simulink model "furnace_emul_v12"  (Simulink 5.0)
settings: Solver=FixedStepDiscrete  StartTime=0.0  StopTime=9000  RelTol=1e-3
values from neighbouring files (symbols this model uses):
  A_amb = pi*(D_e+2*d_ins)*L    (= 0.0498884492)    [tube_ini.m]
  A_e = pi*D_e*L    (= 0.0247557292)    [tube_ini.m]
  A_pi = pi*D_pi*L    (= 0.017592904)    [tube_ini.m]
  A_po = pi*D_po*L    (= 0.0184725492)    [tube_ini.m]
  A_w = pi/4*D_w^2*n_sl    (= 0.0628318)    [tube_ini.m]
  A_wc = pi*D_w*Li    (= 0.01256636)    [tube_ini.m]
  D_pi = D_w+2*DX_R    (= 0.28)    [tube_ini.m]
  D_w = 0.2    [tube_ini.m]
  elem_tmax = 1250    [tube_ini.m]
  F_A_e = lam_p_bct*F_A_e+lam_p_bcb*F_A_e([n:-1:1])    [tube_ini.m]
  F_A_ew = e_ew*A_ew./((1/ei-1)+(1/eo-1)*D_pi/D_w+1./(toeplitz(F1*Li)))    [tube_ini.m]
  F_A_p = lam_p_bct*F_A_p+lam_p_bcb*F_A_p([n:-1:1])    [tube_ini.m]
  F_A_pe = A_ep./((1/ei-1)+(1/eo-1)*D_po/D_e+1./(toeplitz(F1*Li)))    [tube_ini.m]
  F_A_pw = A_pw./((1/ei-1)+(1/eo-1)*D_pi/D_w+1./(toeplitz(F1*Li)))    [tube_ini.m]
  f_amb_ped = 1    [tube_ini.m]
  f_amb_top = .3    (= 0.3)    [tube_ini.m]
  Fb_A_ew = e_ew*Aib./((1/ei-1)+(1/eo-1)*Aib/A+1./(F4*Li))    [tube_ini.m]
  Fb_A_pw = Aib./((1/ei-1)+(1/eo-1)*Aib/A+1./(F4*Li))    [tube_ini.m]
  Fs_e = e_ew*A_e./((1/eo-1)+(1/eo-1)+1./(toeplitz(F5*Li)))    [tube_ini.m]
  Fs_p = A_pi./((1/eo-1)+(1/eo-1)+1./(toeplitz(F5*Li)))    [tube_ini.m]
  gww_bot = ones(N_w,1)*SW    [tube_ini.m]
  gww_top = gww_bot    [tube_ini.m]
  h_amb = 1    [tube_ini.m]
  h_gas = 2    [tube_ini.m]
  H_Z = zeros(n,5)    [tube_ini.m]
  k_adj_ped = 0.6    [tube_ini.m]
  k_adj_top = 0.5    [tube_ini.m]
  L = 0.2    [M_Hist040407.m]    (also in exp303.m = 500:499+ly; tube_ini.m = 0.02)
  lam_p_bcb = 1    [tube_ini.m]
  lam_p_bct = .4    (= 0.4)    [tube_ini.m]
  Li = dx_w    (= 0.02)    [tube_ini.m]
  m_e = rho_e*V_e    (= 0.6312710946)    [tube_ini.m]
  m_p = V_p*rho_p    (= 0.30294980688)    [tube_ini.m]
  m_ped = V_ped*rho_p    (= 1.5079632)    [tube_ini.m]
  m_top = rho_p*V_top    (= 1.5079632)    [tube_ini.m]
  m_w = rho_w*V_w    (= 0.146398094)    [tube_ini.m]
  mcp_adj_ped = 0.36    [tube_ini.m]
  mcp_adj_top = 0.25    [tube_ini.m]
  n = N_w+N_top+N_ped    [tube_ini.m]
  N_ped = round(DX_P/Li)    [tube_ini.m]
  N_top = n-N_w-N_p    [s_tubew.m]    (also in tube_ini.m = round(DX_T/Li))
  N_w = 100/n_sl    (= 50)    [tube_ini.m]
  pow_pm = pow_pml*pi*D_e*n*L/(d_e+d_g)    [tube_ini.m]
  pr_gas = 0.2    [tube_ini.m]
  PRG = 0*SPE; for ii=1:length(profile_loc); PRG(ii,profile_loc(ii))=1;end    [tube_ini.m]
  profile_loc = [N_top,h_zones(1)+round(h_zones(2)/2),   sum(h_zones(1:2))+round(h_zones(3)/2),sum(h_zones(1:3))+round(h_zones(4)/2),   n-N_ped]    [tube_ini.m]
  PRT = PRT'    [tube_ini.m]
  PRW = PRW'    [tube_ini.m]
  SPE = SPE'    [tube_ini.m]
  spike_loc = [round(h_zones(1)/2),h_zones(1)+round(h_zones(2)/2),   sum(h_zones(1:2))+round(h_zones(3)/2),sum(h_zones(1:3))+round(h_zones(4)/2),   sum(h_zones(1:4))+round(h_zones(5)/2)]    [tube_ini.m]
  SPT = SPT'    [tube_ini.m]
  T_0 = T_01*ones(n,1)    [tube_ini.m]
  T_a0 = T_a01*ones(n,1)    [tube_ini.m]
  T_amb = 25    [tube_ini.m]
  T_w0 = T_amb*ones(N_w,1)    [tube_ini.m]
  T_w0_ped = T_amb*ones(N_ped,1)    [tube_ini.m]
  T_w0_top = T_01*ones(N_top,1)    [tube_ini.m]
  Tsa = .5    (= 0.5)    [tube_ini.m]
  tube_tmax = 1200    [tube_ini.m]
  V_a = pi/4*D_pi^2*L    (= 0.00123150328)    [tube_ini.m]
undefined symbols (not defined in the file or in its folder): N, s_tubew
libraries: simulink3 x19, simulink x2
(part 2 of 2)

== system furnace_emul_v12/Furnace Emulator v1.2/Heat Exchange/gas-waf_exch/i-i convection ==
  ta_t0 : Inport
  tw : Inport  Port=2
  Index : Inport  Port=3
  A : Inport  Port=4
  Assignment : Assignment  ElementSrc=External
  Assignment1 : Assignment  ElementSrc=External
  Proportional2 : Gain  Gain=0  SaturateOnIntegerOverflow=on
  Selector1 : Selector  ElementSrc=External  Elements=[1:n]  InputPortWidth=n*2
  Selector3 : Selector  Elements=[1:n]  InputPortWidth=n*2
  convection1 : Subsystem
  dh_a : Outport
  dh_w : Outport  Port=2
  wires:
  Index/1 -> Assignment/3, Selector1/2, Assignment1/3
  Assignment/1 -> convection1/2(T+)
  ta_t0/1 -> convection1/1(T-), Assignment/1, Proportional2/1
  tw/1 -> Assignment/2
  Selector1/1 -> dh_w/1
  convection1/1(Out1) -> Selector3/1, Selector1/1
  Selector3/1 -> dh_a/1
  Assignment1/1 -> convection1/3(A)
  Proportional2/1 -> Assignment1/1
  A/1 -> Assignment1/2

== system furnace_emul_v12/Furnace Emulator v1.2/Heat Exchange/gas-waf_exch/i-i convection1 ==
  ta_t0 : Inport
  tw : Inport  Port=2
  Index : Inport  Port=3
  A : Inport  Port=4
  Assignment : Assignment  ElementSrc=External
  Assignment1 : Assignment  ElementSrc=External
  Proportional2 : Gain  Gain=0  SaturateOnIntegerOverflow=on
  Selector1 : Selector  ElementSrc=External  Elements=[1:n]  InputPortWidth=n*2
  Selector3 : Selector  Elements=[1:n]  InputPortWidth=n*2
  convection1 : Subsystem
  dh_a : Outport
  dh_w : Outport  Port=2
  wires:
  A/1 -> Assignment1/2
  Proportional2/1 -> Assignment1/1
  Assignment1/1 -> convection1/3(A)
  Selector3/1 -> dh_a/1
  convection1/1(Out1) -> Selector1/1, Selector3/1
  Selector1/1 -> dh_w/1
  tw/1 -> Assignment/2
  ta_t0/1 -> Proportional2/1, Assignment/1, convection1/1(T-)
  Assignment/1 -> convection1/2(T+)
  Index/1 -> Assignment1/3, Selector1/2, Assignment/3

== system furnace_emul_v12/Furnace Emulator v1.2/Heat Exchange/prof-waf_xch/waf_rad ==
  Tp+ : Inport  Orientation=left
  Tw- : Inport  Orientation=left  Port=2
  nw0 : Inport  Port=3
  Constant1 : Constant  Value=ones(1,2*n)  VectorParams1D=off
  Constant2 : Constant  Value=ones(2*n,1)  VectorParams1D=off
  MATLAB Fcn : MATLABFcn  MATLABFcn=s_tubew(u,n,N_w,N_ped,F_A_pw,Fb_A_pw,Fs_p)  OutputDimensions=[2*n,2*n]  Output1D=off
  Product : Product  SaturateOnIntegerOverflow=on  InputSameDT=on
  Product{1..4} (4 alike) : Product  Multiplication=Matrix(*)  SaturateOnIntegerOverflow=on  InputSameDT=on
  Reshape : simulink3/Signals & Systems/Reshape  OutputDimensionality=Column vector  OutputDimensions=[N,N_w]
  Reshape1 : simulink3/Signals & Systems/Reshape  OutputDimensionality=Row vector  OutputDimensions=[N,N_w]
  Reshape2 : simulink3/Signals & Systems/Reshape  OutputDimensionality=1-D array  OutputDimensions=[N,N_w]
  Reshape3 : simulink3/Signals & Systems/Reshape  OutputDimensionality=1-D array  OutputDimensions=[N,N_w]
  elem_prof_rad : Subsystem
  dh+ : Outport  Orientation=left
  dh- : Outport  Orientation=left  Port=2
  wires:
  nw0/1 -> MATLAB Fcn/1
  Constant1/1 -> Product1/2, Product4/1
  Reshape/1 -> Product1/1
  Constant2/1 -> Product3/2, Product2/1
  Reshape1/1 -> Product2/2
  Product1/1 -> elem_prof_rad/1(T+)
  Product2/1 -> elem_prof_rad/2(T-)
  MATLAB Fcn/1 -> Product/1
  elem_prof_rad/1(DTH) -> Product/2
  Product/1 -> Product3/1, Product4/2
  Product3/1 -> Reshape2/1
  Product4/1 -> Reshape3/1
  Tp+/1 -> Reshape/1
  Tw-/1 -> Reshape1/1
  Reshape3/1 -> dh-/1
  Reshape2/1 -> dh+/1

== system furnace_emul_v12/Furnace Emulator v1.2/Heat Exchange/profile/amb_prof_rad ==
  T+ : Inport
  T- : Inport  Port=2
  Constant1 : Constant  Value=4
  Constant2 : Constant  Value=273
  Constant3 : Constant  Value=4
  Constant4 : Constant  Value=273
  Math Function : Math  Operator=pow
  Math Function1 : Math  Operator=pow
  Proportional1 : Gain  Gain=5.675  SaturateOnIntegerOverflow=on
  Proportional3 : Gain  Gain=0.01  SaturateOnIntegerOverflow=on
  Proportional4 : Gain  Gain=0.01  SaturateOnIntegerOverflow=on
  Sum1 : Sum  Inputs=2  SaturateOnIntegerOverflow=on  InputSameDT=on
  Sum2 : Sum  Inputs=2  SaturateOnIntegerOverflow=on  InputSameDT=on
  Sum3 : Sum  Inputs=+-  SaturateOnIntegerOverflow=on  InputSameDT=on
  DTH : Outport
  wires:
  Sum3/1 -> Proportional1/1
  Proportional1/1 -> DTH/1
  Math Function1/1 -> Sum3/2
  Math Function/1 -> Sum3/1
  T-/1 -> Sum1/1
  Constant4/1 -> Sum1/2
  Sum1/1 -> Proportional4/1
  Proportional4/1 -> Math Function1/1
  Constant3/1 -> Math Function1/2
  T+/1 -> Sum2/1
  Constant2/1 -> Sum2/2
  Sum2/1 -> Proportional3/1
  Proportional3/1 -> Math Function/1
  Constant1/1 -> Math Function/2

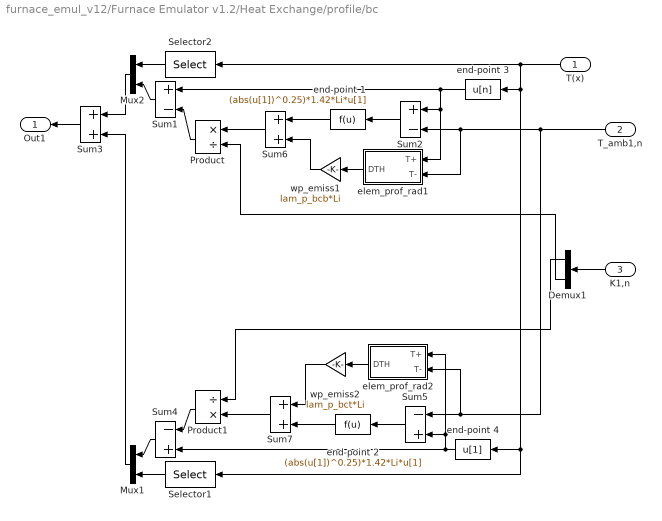
== system furnace_emul_v12/Furnace Emulator v1.2/Heat Exchange/profile/bc ==
  T(x) : Inport  Orientation=left
  T_amb1,n : Inport  Orientation=left  Port=2
  K1,n : Inport  Orientation=left  Port=3
  Demux1 : Demux  Orientation=left  Outputs=2
  Mux1 : Mux  Orientation=left  Inputs=2
  Mux2 : Mux  Orientation=left  Inputs=2
  Product : Product  Orientation=left  Inputs=*/  SaturateOnIntegerOverflow=on  InputSameDT=on
  Product1 : Product  Orientation=left  Inputs=/*  SaturateOnIntegerOverflow=on  InputSameDT=on
  Selector1 : Selector  Orientation=left  Elements=[1:n-1]  InputPortWidth=n
  Selector2 : Selector  Orientation=left  Elements=[2:n]  InputPortWidth=n
  Sum1 : Sum  Orientation=left  Inputs=+-  SaturateOnIntegerOverflow=on  InputSameDT=on
  Sum2 : Sum  Orientation=left  Inputs=+-  SaturateOnIntegerOverflow=on  InputSameDT=on
  Sum3 : Sum  Orientation=left  Inputs=2  SaturateOnIntegerOverflow=on  InputSameDT=on
  Sum4 : Sum  Orientation=left  Inputs=-+  SaturateOnIntegerOverflow=on  InputSameDT=on
  Sum5 : Sum  Orientation=left  Inputs=-+  SaturateOnIntegerOverflow=on  InputSameDT=on
  Sum6 : Sum  Orientation=left  Inputs=2  SaturateOnIntegerOverflow=on  InputSameDT=on
  Sum7 : Sum  Orientation=left  Inputs=2  SaturateOnIntegerOverflow=on  InputSameDT=on
  elem_prof_rad1 : Subsystem  Orientation=left
  elem_prof_rad2 : Subsystem  Orientation=left
  end-point 1 : Fcn  Orientation=left  Expr=(abs(u[1])^0.25)*1.42*Li*u[1]
  end-point 2 : Fcn  Orientation=left  Expr=(abs(u[1])^0.25)*1.42*Li*u[1]
  end-point 3 : Fcn  Orientation=left  Expr=u[n]
  end-point 4 : Fcn  Orientation=left  Expr=u[1]
  wp_emiss1 : Gain  Orientation=left  Gain=lam_p_bcb*Li  SaturateOnIntegerOverflow=on
  wp_emiss2 : Gain  Orientation=left  Gain=lam_p_bct*Li  SaturateOnIntegerOverflow=on
  Out1 : Outport  Orientation=left
  wires:
  Demux1/1 -> Product1/1
  Product1/1 -> Sum4/1
  Demux1/2 -> Product/2
  Product/1 -> Sum1/2
  K1,n/1 -> Demux1/1
  Selector2/1 -> Mux2/1
  Selector1/1 -> Mux1/2
  T(x)/1 -> Selector2/1, end-point 3/1, end-point 4/1, Selector1/1
  Mux1/1 -> Sum3/2
  Mux2/1 -> Sum3/1
  Sum3/1 -> Out1/1
  Sum1/1 -> Mux2/2
  end-point 3/1 -> Sum1/1, Sum2/1, elem_prof_rad1/1(T+)
  Sum2/1 -> end-point 1/1
  Sum4/1 -> Mux1/1
  end-point 4/1 -> Sum4/2, Sum5/2, elem_prof_rad2/1(T+)
  Sum5/1 -> end-point 2/1
  T_amb1,n/1 -> Sum2/2, elem_prof_rad1/2(T-), Sum5/1, elem_prof_rad2/2(T-)
  elem_prof_rad1/1(DTH) -> wp_emiss1/1
  Sum6/1 -> Product/1
  end-point 1/1 -> Sum6/1
  wp_emiss1/1 -> Sum6/2
  elem_prof_rad2/1(DTH) -> wp_emiss2/1
  end-point 2/1 -> Sum7/2
  wp_emiss2/1 -> Sum7/1
  Sum7/1 -> Product1/2

== system furnace_emul_v12/Furnace Emulator v1.2/Heat Exchange/wafer/Top plate ==
  heat In1 : Inport
  amb : Inport  Orientation=left  Port=2
  Constant1 : Constant  Orientation=left  Value=mcp_adj_top
  Constant2 : Constant  Orientation=left  Value=k_adj_top
  Discrete-Time Integrator : DiscreteIntegrator  InitialCondition=T_w0_top  SampleTime=Tsa
  Product : Product  Inputs=*//  SaturateOnIntegerOverflow=on  InputSameDT=on
  Product1 : Product  Inputs=3  SaturateOnIntegerOverflow=on  InputSameDT=on
  Proportional12 : Gain  Orientation=left  Gain=V_top/Li/Li  SaturateOnIntegerOverflow=on
  Proportional2 : Gain  Gain=1/m_top  SaturateOnIntegerOverflow=on
  Proportional7 : Gain  Orientation=left  Gain=2  SaturateOnIntegerOverflow=on
  Selector1 : Selector  Orientation=left  Elements=[1]  InputPortWidth=N_top
  Sum2 : Sum  SaturateOnIntegerOverflow=on  InputSameDT=on
  Sum7 : Sum  Orientation=left  Inputs=-+  SaturateOnIntegerOverflow=on  InputSameDT=on
  bc : Subsystem  Orientation=left
  cp Look-Up Table : Lookup  Orientation=left  InputValues=[400, 600, 800, 1000, 1200]-273  OutputValues=[790 867 913 946 967]  SaturateOnIntegerOverflow=on
  k Look-Up Table : Lookup  Orientation=left  InputValues=[400, 600, 800, 1300]-273  OutputValues="[7.6  5  4.2  3.2 ]"  SaturateOnIntegerOverflow=on
  Ti(x) : Outport
  wires:
  Discrete-Time Integrator/1 -> cp Look-Up Table/1, Ti(x)/1, Proportional7/1, bc/1(T(x)), k Look-Up Table/1
  Sum2/1 -> Proportional2/1
  Product/1 -> Discrete-Time Integrator/1
  Proportional2/1 -> Product/1
  cp Look-Up Table/1 -> Product/2
  heat In1/1 -> Sum2/1
  k Look-Up Table/1 -> Selector1/1, Product1/1
  Selector1/1 -> bc/3(K,1)
  Sum7/1 -> Proportional12/1
  bc/1(Out1) -> Sum7/2
  Proportional7/1 -> Sum7/1
  amb/1 -> bc/2(T_amb1)
  Product1/1 -> Sum2/2
  Proportional12/1 -> Product1/2
  Constant1/1 -> Product/3
  Constant2/1 -> Product1/3

== system furnace_emul_v12/Furnace Emulator v1.2/Heat Exchange/wafer/pedestal ==
  heat In1 : Inport
  Tamb_b : Inport  Orientation=left  Port=2
  Constant1 : Constant  Orientation=left  Value=mcp_adj_ped
  Constant2 : Constant  Orientation=left  Value=k_adj_ped
  Discrete-Time Integrator : DiscreteIntegrator  InitialCondition=T_w0_ped  SampleTime=Tsa
  Product : Product  Inputs=*//  SaturateOnIntegerOverflow=on  InputSameDT=on
  Product1 : Product  Inputs=3  SaturateOnIntegerOverflow=on  InputSameDT=on
  Proportional12 : Gain  Orientation=left  Gain=V_ped/Li/Li  SaturateOnIntegerOverflow=on
  Proportional2 : Gain  Gain=1/m_ped  SaturateOnIntegerOverflow=on
  Proportional7 : Gain  Orientation=left  Gain=2  SaturateOnIntegerOverflow=on
  Selector1 : Selector  Orientation=left  Elements=[N_ped]  InputPortWidth=N_ped
  Sum2 : Sum  SaturateOnIntegerOverflow=on  InputSameDT=on
  Sum7 : Sum  Orientation=left  Inputs=-+  SaturateOnIntegerOverflow=on  InputSameDT=on
  bc : Subsystem  Orientation=left
  cp Look-Up Table : Lookup  Orientation=left  InputValues=[400, 600, 800, 1000, 1200]-273  OutputValues=[790 867 913 946 967]  SaturateOnIntegerOverflow=on
  k Look-Up Table : Lookup  Orientation=left  InputValues=[400, 600, 800, 1300]-273  OutputValues="[7.6  5  4.2  3.2 ]"  SaturateOnIntegerOverflow=on
  Ti(x) : Outport
  wires:
  heat In1/1 -> Sum2/1
  cp Look-Up Table/1 -> Product/2
  Proportional2/1 -> Product/1
  Product/1 -> Discrete-Time Integrator/1
  Sum2/1 -> Proportional2/1
  Discrete-Time Integrator/1 -> cp Look-Up Table/1, Ti(x)/1, Proportional7/1, bc/1(T(x)), k Look-Up Table/1
  k Look-Up Table/1 -> Selector1/1, Product1/2
  Selector1/1 -> bc/3(K,n)
  Sum7/1 -> Proportional12/1
  bc/1(Out1) -> Sum7/2
  Proportional7/1 -> Sum7/1
  Tamb_b/1 -> bc/2(T_ambn)
  Product1/1 -> Sum2/2
  Proportional12/1 -> Product1/1
  Constant1/1 -> Product/3
  Constant2/1 -> Product1/3

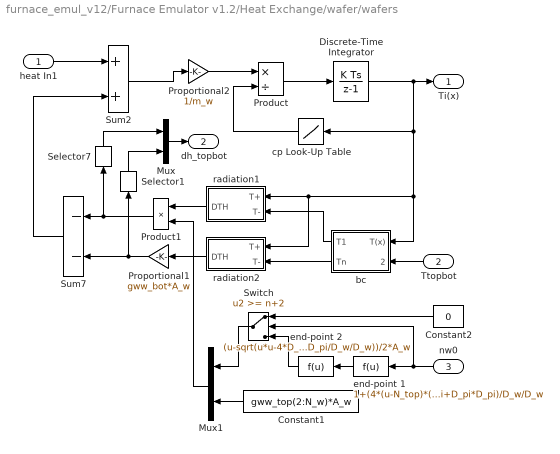
== system furnace_emul_v12/Furnace Emulator v1.2/Heat Exchange/wafer/wafers ==
  heat In1 : Inport
  Ttopbot : Inport  Orientation=left  Port=2
  nw0 : Inport  Orientation=left  Port=3
  Constant1 : Constant  Orientation=left  Value=gww_top(2:N_w)*A_w
  Constant2 : Constant  Orientation=left  Value=0
  Discrete-Time Integrator : DiscreteIntegrator  InitialCondition=T_w0  SampleTime=Tsa
  Mux : Mux  Inputs=2
  Mux1 : Mux  Orientation=left  Inputs=2
  Product : Product  Inputs=*/  SaturateOnIntegerOverflow=on  InputSameDT=on
  Product1 : Product  Orientation=left  SaturateOnIntegerOverflow=on  InputSameDT=on
  Proportional1 : Gain  Orientation=left  Gain=gww_bot*A_w  SaturateOnIntegerOverflow=on
  Proportional2 : Gain  Gain=1/m_w  SaturateOnIntegerOverflow=on
  Selector1 : Selector  Orientation=up  Elements=N_w  InputPortWidth=N_w
  Selector7 : Selector  Orientation=up  InputPortWidth=N_w
  Sum2 : Sum  SaturateOnIntegerOverflow=on  InputSameDT=on
  Sum7 : Sum  Orientation=left  Inputs=--  SaturateOnIntegerOverflow=on  InputSameDT=on
  Switch : Switch  Orientation=left  Threshold=n+2  SaturateOnIntegerOverflow=on  InputSameDT=on
  bc : Subsystem  Orientation=left
  cp Look-Up Table : Lookup  Orientation=left  InputValues=[400, 600, 800, 1000, 1200]-273  OutputValues=[790 867 913 946 967]  SaturateOnIntegerOverflow=on
  end-point 1 : Fcn  Orientation=left  Expr=1+(4*(u-N_top)*(u-N_top)*Li*Li+D_pi*D_pi)/D_w/D_w
  end-point 2 : Fcn  Orientation=left  Expr=(u-sqrt(u*u-4*D_pi*D_pi/D_w/D_w))/2*A_w
  radiation1 : Subsystem  Orientation=left
  radiation2 : Subsystem  Orientation=left
  Ti(x) : Outport
  dh_topbot : Outport  Port=2
  wires:
  Ttopbot/1 -> bc/2(Ttopbot)
  heat In1/1 -> Sum2/1
  Proportional1/1 -> Sum7/2, Selector1/1
  Product1/1 -> Sum7/1, Selector7/1
  cp Look-Up Table/1 -> Product/2
  Proportional2/1 -> Product/1
  Product/1 -> Discrete-Time Integrator/1
  radiation2/1(DTH) -> Proportional1/1
  Sum2/1 -> Proportional2/1
  Discrete-Time Integrator/1 -> Ti(x)/1, radiation2/1(T+), radiation1/1(T+), bc/1(T(x)), cp Look-Up Table/1
  Sum7/1 -> Sum2/2
  bc/1(T1) -> radiation1/2(T-)
  bc/2(Tn) -> radiation2/2(T-)
  Mux/1 -> dh_topbot/1
  radiation1/1(DTH) -> Product1/1
  nw0/1 -> end-point 1/1, Switch/2
  end-point 1/1 -> end-point 2/1
  Constant1/1 -> Mux1/2
  Mux1/1 -> Product1/2
  Selector7/1 -> Mux/1
  Selector1/1 -> Mux/2
  end-point 2/1 -> Switch/3
  Switch/1 -> Mux1/1
  Constant2/1 -> Switch/1

== system furnace_emul_v12/Furnace Emulator v1.2/Heat Exchange/elem-waf_xch/waf_rad/elem_prof_rad ==
  T+ : Inport
  T- : Inport  Port=2
  Constant1 : Constant  Value=4
  Constant2 : Constant  Value=273
  Constant3 : Constant  Value=4
  Constant4 : Constant  Value=273
  Math Function : Math  Operator=pow
  Math Function1 : Math  Operator=pow
  Proportional1 : Gain  Gain=5.675  SaturateOnIntegerOverflow=on
  Proportional3 : Gain  Gain=0.01  SaturateOnIntegerOverflow=on
  Proportional4 : Gain  Gain=0.01  SaturateOnIntegerOverflow=on
  Sum1 : Sum  Inputs=2  SaturateOnIntegerOverflow=on  InputSameDT=on
  Sum2 : Sum  Inputs=2  SaturateOnIntegerOverflow=on  InputSameDT=on
  Sum3 : Sum  Inputs=+-  SaturateOnIntegerOverflow=on  InputSameDT=on
  DTH : Outport
  wires:
  Constant1/1 -> Math Function/2
  Proportional3/1 -> Math Function/1
  Sum2/1 -> Proportional3/1
  Constant2/1 -> Sum2/2
  T+/1 -> Sum2/1
  Constant3/1 -> Math Function1/2
  Proportional4/1 -> Math Function1/1
  Sum1/1 -> Proportional4/1
  Constant4/1 -> Sum1/2
  T-/1 -> Sum1/1
  Math Function/1 -> Sum3/1
  Math Function1/1 -> Sum3/2
  Proportional1/1 -> DTH/1
  Sum3/1 -> Proportional1/1

== system furnace_emul_v12/Furnace Emulator v1.2/Heat Exchange/gas-waf_exch/i-i convection/convection1 ==
  T- : Inport  Orientation=left
  T+ : Inport  Orientation=left  Port=2
  A : Inport  Orientation=left  Port=3
  Abs : Abs  Orientation=left  SaturateOnIntegerOverflow=on
  Constant1 : Constant  Orientation=left  Value=1.3
  Constant3 : Constant  Value=0.25
  Math Function : Math  Orientation=left  Operator=pow
  Product : Product  Orientation=left  Inputs=4  SaturateOnIntegerOverflow=on  InputSameDT=on
  Proportional1 : Gain  Orientation=left  SaturateOnIntegerOverflow=on
  Proportional3 : Gain  Orientation=left  Gain=h_gas  SaturateOnIntegerOverflow=on
  Proportional4 : Gain  Orientation=left  Gain=1.1  SaturateOnIntegerOverflow=on
  Relational Operator : RelationalOperator  Orientation=left  Operator=<  InputSameDT=on
  Sum1 : Sum  Orientation=left  Inputs=2  SaturateOnIntegerOverflow=on  InputSameDT=on
  Sum3 : Sum  Orientation=left  Inputs=-+  SaturateOnIntegerOverflow=on  InputSameDT=on
  Out1 : Outport  Orientation=left
  wires:
  Sum1/1 -> Product/3
  Constant1/1 -> Sum1/1
  Proportional4/1 -> Sum1/2
  Relational Operator/1 -> Proportional4/1
  Product/1 -> Proportional3/1
  Math Function/1 -> Product/2
  Constant3/1 -> Math Function/2
  Proportional1/1 -> Math Function/1
  Abs/1 -> Proportional1/1
  Proportional3/1 -> Out1/1
  T+/1 -> Sum3/2, Relational Operator/2
  T-/1 -> Sum3/1, Relational Operator/1
  Sum3/1 -> Product/1, Abs/1
  A/1 -> Product/4

== system furnace_emul_v12/Furnace Emulator v1.2/Heat Exchange/gas-waf_exch/i-i convection1/convection1 ==
  T- : Inport  Orientation=left
  T+ : Inport  Orientation=left  Port=2
  A : Inport  Orientation=left  Port=3
  Abs : Abs  Orientation=left  SaturateOnIntegerOverflow=on
  Constant1 : Constant  Orientation=left  Value=1.3
  Constant3 : Constant  Value=0.25
  Math Function : Math  Orientation=left  Operator=pow
  Product : Product  Orientation=left  Inputs=4  SaturateOnIntegerOverflow=on  InputSameDT=on
  Proportional1 : Gain  Orientation=left  SaturateOnIntegerOverflow=on
  Proportional3 : Gain  Orientation=left  Gain=h_gas  SaturateOnIntegerOverflow=on
  Proportional4 : Gain  Orientation=left  Gain=1.1  SaturateOnIntegerOverflow=on
  Relational Operator : RelationalOperator  Orientation=left  Operator=<  InputSameDT=on
  Sum1 : Sum  Orientation=left  Inputs=2  SaturateOnIntegerOverflow=on  InputSameDT=on
  Sum3 : Sum  Orientation=left  Inputs=-+  SaturateOnIntegerOverflow=on  InputSameDT=on
  Out1 : Outport  Orientation=left
  wires:
  A/1 -> Product/4
  Sum3/1 -> Abs/1, Product/1
  T-/1 -> Relational Operator/1, Sum3/1
  T+/1 -> Relational Operator/2, Sum3/2
  Proportional3/1 -> Out1/1
  Abs/1 -> Proportional1/1
  Proportional1/1 -> Math Function/1
  Constant3/1 -> Math Function/2
  Math Function/1 -> Product/2
  Product/1 -> Proportional3/1
  Relational Operator/1 -> Proportional4/1
  Proportional4/1 -> Sum1/2
  Constant1/1 -> Sum1/1
  Sum1/1 -> Product/3

== system furnace_emul_v12/Furnace Emulator v1.2/Heat Exchange/prof-waf_xch/waf_rad/elem_prof_rad ==
  T+ : Inport
  T- : Inport  Port=2
  Constant1 : Constant  Value=4
  Constant2 : Constant  Value=273
  Constant3 : Constant  Value=4
  Constant4 : Constant  Value=273
  Math Function : Math  Operator=pow
  Math Function1 : Math  Operator=pow
  Proportional1 : Gain  Gain=5.675  SaturateOnIntegerOverflow=on
  Proportional3 : Gain  Gain=0.01  SaturateOnIntegerOverflow=on
  Proportional4 : Gain  Gain=0.01  SaturateOnIntegerOverflow=on
  Sum1 : Sum  Inputs=2  SaturateOnIntegerOverflow=on  InputSameDT=on
  Sum2 : Sum  Inputs=2  SaturateOnIntegerOverflow=on  InputSameDT=on
  Sum3 : Sum  Inputs=+-  SaturateOnIntegerOverflow=on  InputSameDT=on
  DTH : Outport
  wires:
  Sum3/1 -> Proportional1/1
  Proportional1/1 -> DTH/1
  Math Function1/1 -> Sum3/2
  Math Function/1 -> Sum3/1
  T-/1 -> Sum1/1
  Constant4/1 -> Sum1/2
  Sum1/1 -> Proportional4/1
  Proportional4/1 -> Math Function1/1
  Constant3/1 -> Math Function1/2
  T+/1 -> Sum2/1
  Constant2/1 -> Sum2/2
  Sum2/1 -> Proportional3/1
  Proportional3/1 -> Math Function/1
  Constant1/1 -> Math Function/2

== system furnace_emul_v12/Furnace Emulator v1.2/Heat Exchange/profile/bc/elem_prof_rad1 ==
  T+ : Inport
  T- : Inport  Port=2
  Constant1 : Constant  Value=4
  Constant2 : Constant  Value=273
  Constant3 : Constant  Value=4
  Constant4 : Constant  Value=273
  Math Function : Math  Operator=pow
  Math Function1 : Math  Operator=pow
  Proportional1 : Gain  Gain=5.675  SaturateOnIntegerOverflow=on
  Proportional3 : Gain  Gain=0.01  SaturateOnIntegerOverflow=on
  Proportional4 : Gain  Gain=0.01  SaturateOnIntegerOverflow=on
  Sum1 : Sum  Inputs=2  SaturateOnIntegerOverflow=on  InputSameDT=on
  Sum2 : Sum  Inputs=2  SaturateOnIntegerOverflow=on  InputSameDT=on
  Sum3 : Sum  Inputs=+-  SaturateOnIntegerOverflow=on  InputSameDT=on
  DTH : Outport
  wires:
  Sum3/1 -> Proportional1/1
  Proportional1/1 -> DTH/1
  Math Function1/1 -> Sum3/2
  Math Function/1 -> Sum3/1
  T-/1 -> Sum1/1
  Constant4/1 -> Sum1/2
  Sum1/1 -> Proportional4/1
  Proportional4/1 -> Math Function1/1
  Constant3/1 -> Math Function1/2
  T+/1 -> Sum2/1
  Constant2/1 -> Sum2/2
  Sum2/1 -> Proportional3/1
  Proportional3/1 -> Math Function/1
  Constant1/1 -> Math Function/2

== system furnace_emul_v12/Furnace Emulator v1.2/Heat Exchange/profile/bc/elem_prof_rad2 ==
  T+ : Inport
  T- : Inport  Port=2
  Constant1 : Constant  Value=4
  Constant2 : Constant  Value=273
  Constant3 : Constant  Value=4
  Constant4 : Constant  Value=273
  Math Function : Math  Operator=pow
  Math Function1 : Math  Operator=pow
  Proportional1 : Gain  Gain=5.675  SaturateOnIntegerOverflow=on
  Proportional3 : Gain  Gain=0.01  SaturateOnIntegerOverflow=on
  Proportional4 : Gain  Gain=0.01  SaturateOnIntegerOverflow=on
  Sum1 : Sum  Inputs=2  SaturateOnIntegerOverflow=on  InputSameDT=on
  Sum2 : Sum  Inputs=2  SaturateOnIntegerOverflow=on  InputSameDT=on
  Sum3 : Sum  Inputs=+-  SaturateOnIntegerOverflow=on  InputSameDT=on
  DTH : Outport
  wires:
  Constant1/1 -> Math Function/2
  Proportional3/1 -> Math Function/1
  Sum2/1 -> Proportional3/1
  Constant2/1 -> Sum2/2
  T+/1 -> Sum2/1
  Constant3/1 -> Math Function1/2
  Proportional4/1 -> Math Function1/1
  Sum1/1 -> Proportional4/1
  Constant4/1 -> Sum1/2
  T-/1 -> Sum1/1
  Math Function/1 -> Sum3/1
  Math Function1/1 -> Sum3/2
  Proportional1/1 -> DTH/1
  Sum3/1 -> Proportional1/1

== system furnace_emul_v12/Furnace Emulator v1.2/Heat Exchange/wafer/Top plate/bc ==
  T(x) : Inport  Orientation=left
  T_amb1 : Inport  Orientation=left  Port=2
  K,1 : Inport  Port=3
  Mux1 : Mux  Orientation=left  Inputs=2
  Mux2 : Mux  Orientation=left  Inputs=2
  Product : Product  Orientation=left  Inputs=*/  SaturateOnIntegerOverflow=on  InputSameDT=on
  Proportional3 : Gain  Orientation=left  Gain=f_amb_top*Li  SaturateOnIntegerOverflow=on
  Selector1 : Selector  Orientation=left  Elements=[2:N_top]  InputPortWidth=N_top
  Selector2 : Selector  Orientation=left  Elements=[1:N_top-1]  InputPortWidth=N_top
  Sum1 : Sum  Orientation=left  Inputs=+-  SaturateOnIntegerOverflow=on  InputSameDT=on
  Sum2 : Sum  Orientation=left  Inputs=+-  SaturateOnIntegerOverflow=on  InputSameDT=on
  Sum3 : Sum  Orientation=left  Inputs=2  SaturateOnIntegerOverflow=on  InputSameDT=on
  Sum6 : Sum  Orientation=left  Inputs=2  SaturateOnIntegerOverflow=on  InputSameDT=on
  end-point 1 : Fcn  Orientation=left  Expr=(abs(u[1])^0.25)*1.42*Li*u[1]
  end-point 3 : Fcn  Orientation=left  Expr=u[1]
  end-point 4 : Fcn  Orientation=left  Expr=u[N_top]
  radiation1 : Subsystem  Orientation=left
  Out1 : Outport  Orientation=left
  wires:
  Product/1 -> Sum1/2
  K,1/1 -> Product/2
  T(x)/1 -> Selector2/1, end-point 3/1, end-point 4/1, Selector1/1
  Mux1/1 -> Sum3/2
  Mux2/1 -> Sum3/1
  Sum3/1 -> Out1/1
  end-point 3/1 -> Sum1/1, Sum2/1, radiation1/1(T+)
  Sum2/1 -> end-point 1/1
  Sum6/1 -> Product/1
  end-point 1/1 -> Sum6/1
  radiation1/1(DTH) -> Proportional3/1
  Proportional3/1 -> Sum6/2
  T_amb1/1 -> Sum2/2, radiation1/2(T-)
  Selector1/1 -> Mux1/1
  end-point 4/1 -> Mux1/2
  Selector2/1 -> Mux2/2
  Sum1/1 -> Mux2/1

== system furnace_emul_v12/Furnace Emulator v1.2/Heat Exchange/wafer/pedestal/bc ==
  T(x) : Inport  Orientation=left
  T_ambn : Inport  Orientation=left  Port=2
  K,n : Inport  Port=3
  Mux1 : Mux  Orientation=left  Inputs=2
  Mux2 : Mux  Orientation=left  Inputs=2
  Product : Product  Orientation=left  Inputs=*/  SaturateOnIntegerOverflow=on  InputSameDT=on
  Proportional3 : Gain  Orientation=left  Gain=f_amb_ped*Li  SaturateOnIntegerOverflow=on
  Selector1 : Selector  Orientation=left  Elements=[1:N_ped-1]  InputPortWidth=N_ped
  Selector2 : Selector  Orientation=left  Elements=[2:N_ped]  InputPortWidth=N_ped
  Sum1 : Sum  Orientation=left  Inputs=+-  SaturateOnIntegerOverflow=on  InputSameDT=on
  Sum2 : Sum  Orientation=left  Inputs=+-  SaturateOnIntegerOverflow=on  InputSameDT=on
  Sum3 : Sum  Orientation=left  Inputs=2  SaturateOnIntegerOverflow=on  InputSameDT=on
  Sum6 : Sum  Orientation=left  Inputs=2  SaturateOnIntegerOverflow=on  InputSameDT=on
  end-point 1 : Fcn  Orientation=left  Expr=(abs(u[1])^0.25)*1.42*Li*u[1]
  end-point 3 : Fcn  Orientation=left  Expr=u[N_ped]
  end-point 4 : Fcn  Orientation=left  Expr=u[1]
  radiation1 : Subsystem  Orientation=left
  Out1 : Outport  Orientation=left
  wires:
  Product/1 -> Sum1/2
  K,n/1 -> Product/2
  Selector2/1 -> Mux2/1
  Selector1/1 -> Mux1/2
  T(x)/1 -> Selector2/1, end-point 3/1, end-point 4/1, Selector1/1
  Mux1/1 -> Sum3/2
  Mux2/1 -> Sum3/1
  Sum3/1 -> Out1/1
  Sum1/1 -> Mux2/2
  end-point 3/1 -> Sum1/1, Sum2/1, radiation1/1(T+)
  Sum2/1 -> end-point 1/1
  end-point 4/1 -> Mux1/1
  Sum6/1 -> Product/1
  end-point 1/1 -> Sum6/1
  radiation1/1(DTH) -> Proportional3/1
  Proportional3/1 -> Sum6/2
  T_ambn/1 -> Sum2/2, radiation1/2(T-)

== system furnace_emul_v12/Furnace Emulator v1.2/Heat Exchange/wafer/wafers/bc ==
  T(x) : Inport  Orientation=left
  Ttopbot : Inport  Orientation=left  Port=2
  Mux1 : Mux  Orientation=left  Inputs=2
  Mux2 : Mux  Orientation=left  Inputs=2
  Selector1 : Selector  Orientation=left  Elements=[1:N_w-1]  InputPortWidth=N_w
  Selector2 : Selector  Orientation=left  Elements=[2:N_w]  InputPortWidth=N_w
  Selector3 : Selector  Orientation=up  Elements=2  InputPortWidth=2
  Selector4 : Selector  Orientation=down  InputPortWidth=2
  T1 : Outport  Orientation=left
  Tn : Outport  Orientation=left  Port=2
  wires:
  Ttopbot/1 -> Selector3/1, Selector4/1
  Selector2/1 -> Mux2/1
  Selector1/1 -> Mux1/2
  T(x)/1 -> Selector1/1, Selector2/1
  Mux1/1 -> T1/1
  Mux2/1 -> Tn/1
  Selector3/1 -> Mux2/2
  Selector4/1 -> Mux1/1

== system furnace_emul_v12/Furnace Emulator v1.2/Heat Exchange/wafer/wafers/radiation1 ==
  T+ : Inport
  T- : Inport  Port=2
  Constant1 : Constant  Value=4
  Constant2 : Constant  Value=273
  Constant3 : Constant  Value=4
  Constant4 : Constant  Value=273
  Math Function : Math  Operator=pow
  Math Function1 : Math  Operator=pow
  Proportional1 : Gain  Gain=5.675  SaturateOnIntegerOverflow=on
  Proportional3 : Gain  Gain=0.01  SaturateOnIntegerOverflow=on
  Proportional4 : Gain  Gain=0.01  SaturateOnIntegerOverflow=on
  Sum1 : Sum  Inputs=2  SaturateOnIntegerOverflow=on  InputSameDT=on
  Sum2 : Sum  Inputs=2  SaturateOnIntegerOverflow=on  InputSameDT=on
  Sum3 : Sum  Inputs=+-  SaturateOnIntegerOverflow=on  InputSameDT=on
  DTH : Outport
  wires:
  Sum3/1 -> Proportional1/1
  Proportional1/1 -> DTH/1
  Math Function1/1 -> Sum3/2
  Math Function/1 -> Sum3/1
  T-/1 -> Sum1/1
  Constant4/1 -> Sum1/2
  Sum1/1 -> Proportional4/1
  Proportional4/1 -> Math Function1/1
  Constant3/1 -> Math Function1/2
  T+/1 -> Sum2/1
  Constant2/1 -> Sum2/2
  Sum2/1 -> Proportional3/1
  Proportional3/1 -> Math Function/1
  Constant1/1 -> Math Function/2

== system furnace_emul_v12/Furnace Emulator v1.2/Heat Exchange/wafer/wafers/radiation2 ==
  T+ : Inport
  T- : Inport  Port=2
  Constant1 : Constant  Value=4
  Constant2 : Constant  Value=273
  Constant3 : Constant  Value=4
  Constant4 : Constant  Value=273
  Math Function : Math  Operator=pow
  Math Function1 : Math  Operator=pow
  Proportional1 : Gain  Gain=5.675  SaturateOnIntegerOverflow=on
  Proportional3 : Gain  Gain=0.01  SaturateOnIntegerOverflow=on
  Proportional4 : Gain  Gain=0.01  SaturateOnIntegerOverflow=on
  Sum1 : Sum  Inputs=2  SaturateOnIntegerOverflow=on  InputSameDT=on
  Sum2 : Sum  Inputs=2  SaturateOnIntegerOverflow=on  InputSameDT=on
  Sum3 : Sum  Inputs=+-  SaturateOnIntegerOverflow=on  InputSameDT=on
  DTH : Outport
  wires:
  Constant1/1 -> Math Function/2
  Proportional3/1 -> Math Function/1
  Sum2/1 -> Proportional3/1
  Constant2/1 -> Sum2/2
  T+/1 -> Sum2/1
  Constant3/1 -> Math Function1/2
  Proportional4/1 -> Math Function1/1
  Sum1/1 -> Proportional4/1
  Constant4/1 -> Sum1/2
  T-/1 -> Sum1/1
  Math Function/1 -> Sum3/1
  Math Function1/1 -> Sum3/2
  Proportional1/1 -> DTH/1
  Sum3/1 -> Proportional1/1

== system furnace_emul_v12/Furnace Emulator v1.2/Heat Exchange/wafer/Top plate/bc/radiation1 ==
  T+ : Inport
  T- : Inport  Port=2
  Constant1 : Constant  Value=4
  Constant2 : Constant  Value=273
  Constant3 : Constant  Value=4
  Constant4 : Constant  Value=273
  Math Function : Math  Operator=pow
  Math Function1 : Math  Operator=pow
  Proportional1 : Gain  Gain=5.675  SaturateOnIntegerOverflow=on
  Proportional3 : Gain  Gain=0.01  SaturateOnIntegerOverflow=on
  Proportional4 : Gain  Gain=0.01  SaturateOnIntegerOverflow=on
  Sum1 : Sum  Inputs=2  SaturateOnIntegerOverflow=on  InputSameDT=on
  Sum2 : Sum  Inputs=2  SaturateOnIntegerOverflow=on  InputSameDT=on
  Sum3 : Sum  Inputs=+-  SaturateOnIntegerOverflow=on  InputSameDT=on
  DTH : Outport
  wires:
  Sum3/1 -> Proportional1/1
  Proportional1/1 -> DTH/1
  Math Function1/1 -> Sum3/2
  Math Function/1 -> Sum3/1
  T-/1 -> Sum1/1
  Constant4/1 -> Sum1/2
  Sum1/1 -> Proportional4/1
  Proportional4/1 -> Math Function1/1
  Constant3/1 -> Math Function1/2
  T+/1 -> Sum2/1
  Constant2/1 -> Sum2/2
  Sum2/1 -> Proportional3/1
  Proportional3/1 -> Math Function/1
  Constant1/1 -> Math Function/2

== system furnace_emul_v12/Furnace Emulator v1.2/Heat Exchange/wafer/pedestal/bc/radiation1 ==
  T+ : Inport
  T- : Inport  Port=2
  Constant1 : Constant  Value=4
  Constant2 : Constant  Value=273
  Constant3 : Constant  Value=4
  Constant4 : Constant  Value=273
  Math Function : Math  Operator=pow
  Math Function1 : Math  Operator=pow
  Proportional1 : Gain  Gain=5.675  SaturateOnIntegerOverflow=on
  Proportional3 : Gain  Gain=0.01  SaturateOnIntegerOverflow=on
  Proportional4 : Gain  Gain=0.01  SaturateOnIntegerOverflow=on
  Sum1 : Sum  Inputs=2  SaturateOnIntegerOverflow=on  InputSameDT=on
  Sum2 : Sum  Inputs=2  SaturateOnIntegerOverflow=on  InputSameDT=on
  Sum3 : Sum  Inputs=+-  SaturateOnIntegerOverflow=on  InputSameDT=on
  DTH : Outport
  wires:
  Sum3/1 -> Proportional1/1
  Proportional1/1 -> DTH/1
  Math Function1/1 -> Sum3/2
  Math Function/1 -> Sum3/1
  T-/1 -> Sum1/1
  Constant4/1 -> Sum1/2
  Sum1/1 -> Proportional4/1
  Proportional4/1 -> Math Function1/1
  Constant3/1 -> Math Function1/2
  T+/1 -> Sum2/1
  Constant2/1 -> Sum2/2
  Sum2/1 -> Proportional3/1
  Proportional3/1 -> Math Function/1
  Constant1/1 -> Math Function/2
